simulink model "MRsim"  (R2018a)
settings: Solver=ode8  StartTime=0.0  StopTime=20  FixedStep=dt  RelTol=1e-5
values from neighbouring files (symbols this model uses):
  A = 300    [script.m]
  Alpha = alphab + (alphaa - alphab)*exp(-alphac*ic)    [script.m]
  bdg = ss(A1,B,C1,D)    [script.m]
  Beta = betab + (betaa - betab)*exp(-betac*ic)    [script.m]
  C0 = c0b + (c0a - c0b)*exp(-c0c*ic)    [script.m]
  dt = 1/10000    (= 0.0001)    [script.m]
  Gact = 1.6e7/((s+151.7)*(s^2+250.4*s+1.061e5))    [script.m]
  Gamma = Beta    [script.m]
  k0 = 0.0    (= 0)    [script.m]
  k1 = 0.0    (= 0)    [script.m]
undefined symbols (not defined in the file or in its folder): DiscIntNeverNeededParam
settings Model: Creator=amira  LastModifiedBy=amira
settings SolverCC: AlgebraicLoopSolver=LineSearch

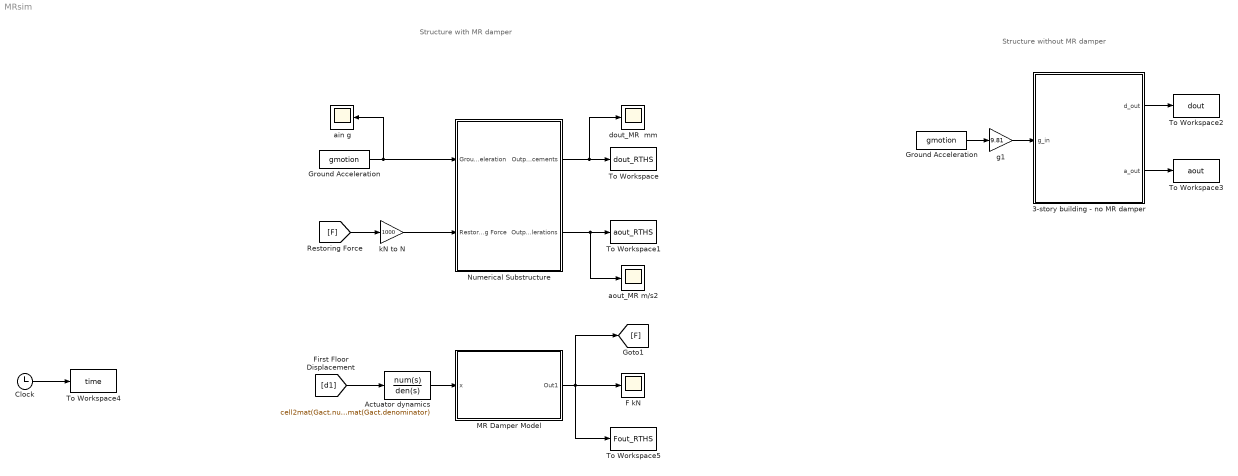
== system MRsim ==
  note: Structure without MR damper
  note: Structure with MR damper
  " Ground Acceleration" : FromWorkspace  VariableName=gmotion  SampleTime=1/200
  3-story building - no MR damper : Subsystem
  Actuator dynamics : TransferFcn  Numerator=cell2mat(Gact.numerator)  Denominator=cell2mat(Gact.denominator)
  Clock : Clock
  F kN : Scope
  Ground Acceleration : FromWorkspace  VariableName=gmotion  SampleTime=1/200
  MR Damper Model : Subsystem
      mask Display: image('C:\Users\amira\Documents\PhD\Developments\12 MR Damper Project\4 MR Damper Model\Picture1.jpg');
  Numerical Substructure : Subsystem
      mask Display: image('C:\Users\amira\Documents\PhD\Developments\12 MR Damper Project\4 MR Damper Model\Building pic.PNG');
  To Workspace : ToWorkspace  VariableName=dout_RTHS  SampleTime=dt
  To Workspace1 : ToWorkspace  VariableName=aout_RTHS  SampleTime=dt
  To Workspace2 : ToWorkspace  VariableName=dout  SampleTime=dt
  To Workspace3 : ToWorkspace  VariableName=aout  SampleTime=dt
  To Workspace4 : ToWorkspace  VariableName=time  SampleTime=dt
  To Workspace5 : ToWorkspace  VariableName=Fout_RTHS  SampleTime=dt
  ain g : Scope
  aout_MR m/s2 : Scope
  dout_MR  mm : Scope
  g1 : Gain  Gain=9.81
  kN to N : Gain  Gain=1000
  wires:
  [F] -> kN to N/1
  Clock/1 -> To Workspace4/1
  [d1] -> Actuator dynamics/1
  Actuator dynamics/1 -> MR Damper Model/1(x)
  MR Damper Model/1(Out1) -> [F], To Workspace5/1, F kN/1
  " Ground Acceleration"/1 -> g1/1
  3-story building - no MR damper/1(d_out) -> To Workspace2/1
  3-story building - no MR damper/2(a_out) -> To Workspace3/1
  g1/1 -> 3-story building - no MR damper/1(g_in)
  Ground Acceleration/1 -> ain g/1, Numerical Substructure/1(Ground Acceleration)
  Numerical Substructure/1(Output Displacements) -> dout_MR  mm/1, To Workspace/1
  Numerical Substructure/2(Output Accelerations) -> To Workspace1/1, aout_MR m/s2/1
  kN to N/1 -> Numerical Substructure/2(Restoring Force)

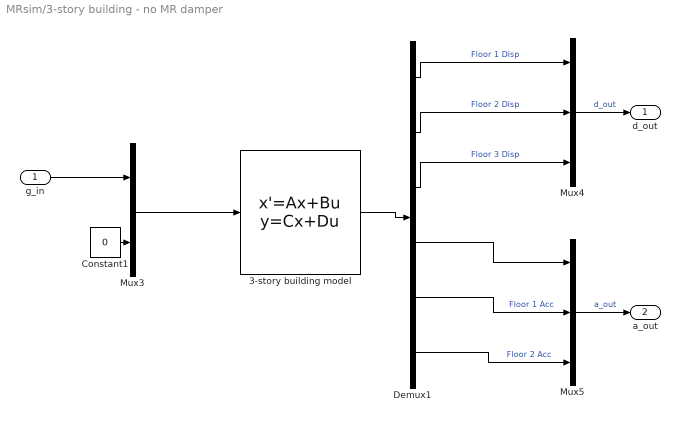
== system MRsim/3-story building - no MR damper ==
  g_in : Inport
  " 3-story building model" : StateSpace  A=bdg.A  B=bdg.B  C=bdg.C  D=bdg.D  InitialCondition=0
  Constant1 : Constant  Value=0
  Demux1 : Demux  Outputs=6
  Mux3 : Mux  Inputs=2
  Mux4 : Mux  Inputs=3
  Mux5 : Mux  Inputs=3
  d_out : Outport
  a_out : Outport  Port=2
  wires:
  Demux1/2 -> Mux4/2  "Floor 2 Disp"
  Demux1/3 -> Mux4/3  "Floor 3 Disp"
  Mux5/1 -> a_out/1  "a_out"
  Demux1/1 -> Mux4/1  "Floor 1 Disp"
  " 3-story building model"/1 -> Demux1/1
  Constant1/1 -> Mux3/2
  Mux3/1 -> " 3-story building model"/1
  g_in/1 -> Mux3/1
  Mux4/1 -> d_out/1  "d_out"
  Demux1/4 -> Mux5/1
  Demux1/5 -> Mux5/2  "Floor 1 Acc"
  Demux1/6 -> Mux5/3  "Floor 2 Acc"

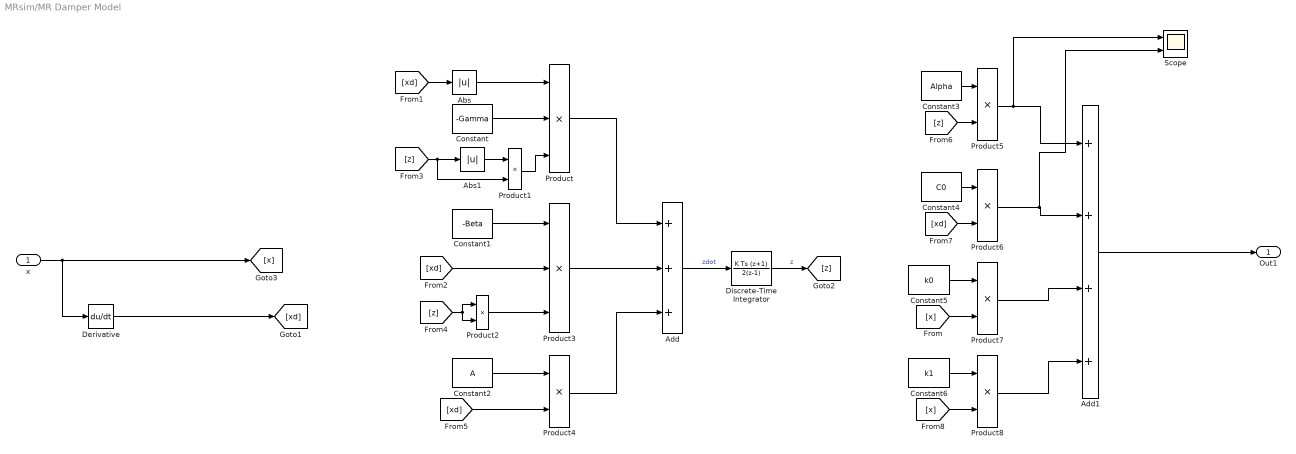
== system MRsim/MR Damper Model ==
  x : Inport
  Abs : Abs
  Abs1 : Abs
  Add : Sum  Inputs=3
  Add1 : Sum  Inputs=4
  Constant : Constant  Value=-Gamma
  Constant1 : Constant  Value=-Beta
  Constant2 : Constant  Value=A
  Constant3 : Constant  Value=Alpha
  Constant4 : Constant  Value=C0
  Constant5 : Constant  Value=k0
  Constant6 : Constant  Value=k1
  Derivative : Derivative
  Discrete-Time Integrator : DiscreteIntegrator  IntegratorMethod=Integration: Trapezoidal  SampleTime=dt  ICPrevOutput=DiscIntNeverNeededParam  ICPrevScaledInput=DiscIntNeverNeededParam
  Product : Product  Inputs=3
  Product{1..2,4..8} (7 alike) : Product
  Product3 : Product  Inputs=3
  Scope : Scope  NumInputPorts=2
  Out1 : Outport
  wires:
  [xd] -> Abs/1
  Product3/1 -> Add/2
  [xd] -> Product3/2
  [z] -> Product2/2, Product2/1
  Constant4/1 -> Product6/1
  Product/1 -> Add/1
  [xd] -> Product6/2
  Add1/1 -> Out1/1
  [xd] -> Product4/2
  [z] -> Product1/2, Abs1/1
  Product4/1 -> Add/3
  Constant/1 -> Product/2
  Constant3/1 -> Product5/1
  Abs1/1 -> Product1/1
  Constant6/1 -> Product8/1
  Product6/1 -> Scope/2, Add1/2
  Product8/1 -> Add1/4
  Constant5/1 -> Product7/1
  Product7/1 -> Add1/3
  Product5/1 -> Scope/1, Add1/1
  [x] -> Product7/2
  Product1/1 -> Product/3
  Constant2/1 -> Product4/1
  Add/1 -> Discrete-Time Integrator/1  "zdot"
  Discrete-Time Integrator/1 -> [z]  "z"
  [x] -> Product8/2
  [z] -> Product5/2
  Constant1/1 -> Product3/1
  Product2/1 -> Product3/3
  Abs/1 -> Product/1
  x/1 -> Derivative/1, [x]
  Derivative/1 -> [xd]

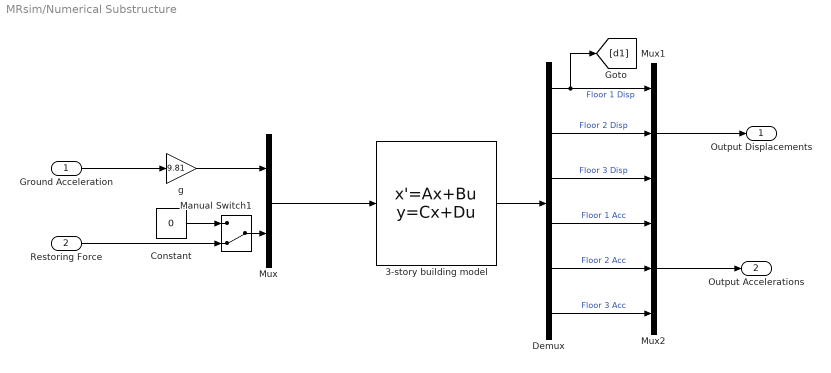
== system MRsim/Numerical Substructure ==
  Ground Acceleration : Inport
  Restoring Force : Inport  Port=2
  3-story building model : StateSpace  A=bdg.A  B=bdg.B  C=bdg.C  D=bdg.D  InitialCondition=0
  Constant : Constant  Value=0
  Demux : Demux  Outputs=6
  Manual Switch1 : ManualSwitch  CurrentSetting=0
  Mux : Mux  Inputs=2
  Mux1 : Mux  Inputs=3
  Mux2 : Mux  Inputs=3
  g : Gain  Gain=9.81
  Output Displacements : Outport
  Output Accelerations : Outport  Port=2
  wires:
  3-story building model/1 -> Demux/1
  Demux/1 -> Mux1/1, [d1]  "Floor 1 Disp"
  g/1 -> Mux/1
  Constant/1 -> Manual Switch1/1
  Demux/3 -> Mux1/3  "Floor 3 Disp"
  Manual Switch1/1 -> Mux/2
  Mux/1 -> 3-story building model/1
  Demux/4 -> Mux2/1  "Floor 1 Acc"
  Demux/5 -> Mux2/2  "Floor 2 Acc"
  Mux2/1 -> Output Accelerations/1
  Demux/2 -> Mux1/2  "Floor 2 Disp"
  Demux/6 -> Mux2/3  "Floor 3 Acc"
  Restoring Force/1 -> Manual Switch1/2
  Mux1/1 -> Output Displacements/1
  Ground Acceleration/1 -> g/1
